simulink model "PID"  (R2015a)
settings: Solver=ode45  StartTime=0.0  StopTime=10.0  RelTol=1e-3
undefined symbols (not defined in the file): g, k, k1, k2, l, m
settings Model: SimulationMode=accelerator  Creator=Benjamin Nicolas  LastModifiedBy=Benjamin Nicolas

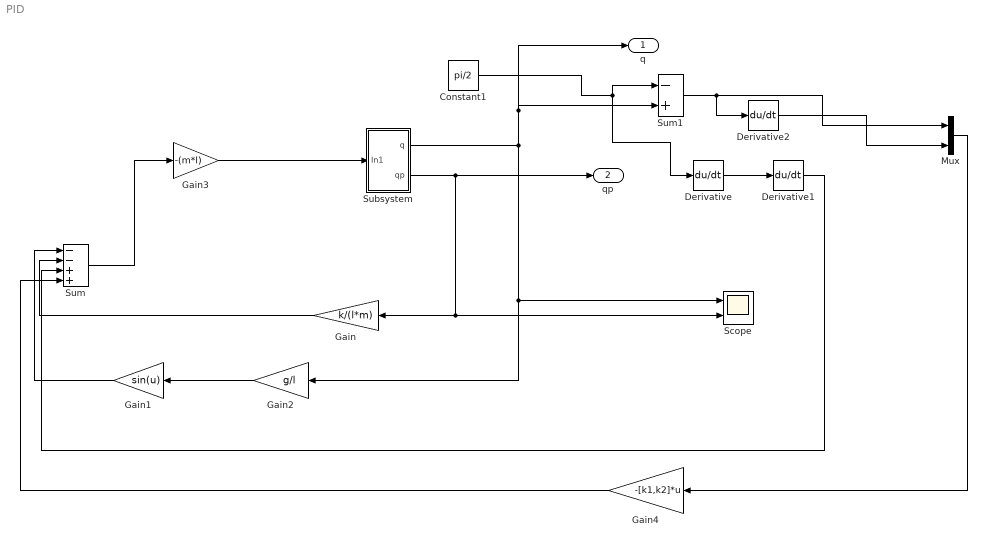
== system PID ==
  Constant1 : Constant  Value=pi/2
  Derivative : Derivative
  Derivative1 : Derivative
  Derivative2 : Derivative
  Gain : Gain  Gain=k/(l*m)
  Gain1 : Gain  Gain=sin(u)
  Gain2 : Gain  Gain=g/l
  Gain3 : Gain  Gain=-(m*l)
  Gain4 : Gain  Gain=-[k1,k2]*u
  Mux : Mux  Inputs=2
  Scope : Scope  NumInputPorts=2
      settings: YMin=-5~-5  YMax=5~5
  Subsystem : Subsystem
  Sum : Sum  Inputs=|--++
  Sum1 : Sum  Inputs=|-+
  "q " : Outport
  "qp " : Outport  Port=2
  wires:
  Subsystem/1("q ") -> Scope/1, Gain2/1, Sum1/2, "q "/1
  Subsystem/2("qp ") -> Scope/2, Gain/1, "qp "/1
  Constant1/1 -> Derivative/1, Sum1/1
  Gain3/1 -> Subsystem/1(In1)
  Sum/1 -> Gain3/1
  Gain/1 -> Sum/2
  Derivative/1 -> Derivative1/1
  Sum1/1 -> Mux/1, Derivative2/1
  Derivative2/1 -> Mux/2
  Gain1/1 -> Sum/1
  Gain2/1 -> Gain1/1
  Derivative1/1 -> Sum/3
  Mux/1 -> Gain4/1
  Gain4/1 -> Sum/4

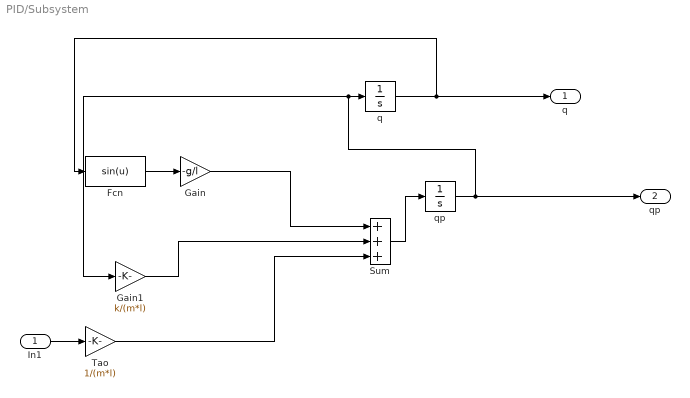
== system PID/Subsystem ==
  In1 : Inport
  Fcn : Fcn  Expr=sin(u)
  Gain : Gain  Gain=-g/l
  Gain1 : Gain  Gain=k/(m*l)
  Sum : Sum  Inputs=+++
  "Tao " : Gain  Gain=1/(m*l)
  q : Integrator
  qp : Integrator
  "q " : Outport
  "qp " : Outport  Port=2
  wires:
  Sum/1 -> qp/1
  In1/1 -> "Tao "/1
  Gain1/1 -> Sum/2
  Gain/1 -> Sum/1
  q/1 -> "q "/1, Fcn/1
  Fcn/1 -> Gain/1
  qp/1 -> "qp "/1, q/1, Gain1/1
  "Tao "/1 -> Sum/3
